simulink model "DualStreamSSR"  (R2023a)
(part 5 of 6)

  filter6 : aieBasic/AIE Class Kernel  KernelAllAttrs=|  PortNames={'sin1'; 'sin2'; 'cin'; 'cout'}  PortSerializedTypes={'{Q2{P{Tinput_stream{1{t{Scint16}}}}}}'; '{Q2{P{Tinput_stream{1{t{Scint16}}}}}}'; '{P{Tinput_stream{1{t{Scacc48_t}}}}}'; '{P{Toutput_stream{1{t{Scacc48_t}}}}}'}  PortWindowSizes={0.000000000000000000e+00; 0.000000000000000000e+00; 0.000000000000000000e+00; 0.000000000000000000e+00}  PortWindowMargins={0.000000000000000000e+00; 0.000000000000000000e+00; 0.000000000000000000e+00; 0.000000000000000000e+00}  PortSynchronicities={'auto', 'auto', 'auto', 'auto'}  PortSignalSizes={0.000000000000000000e+00; 0.000000000000000000e+00; 0.000000000000000000e+00; 8.000000000000000000e+00}  ClassTemplateSpecKind=implicit  ClassTemplateParamNames={'NSamples'; 'ShiftAcc'; 'DiscardSample'; 'SwapRead'}  ClassTemplateParamKinds={'nontype'; 'nontype'; 'nontype'; 'nontype'}  ClassTemplateParamTypes={'int'; 'int'; 'bool'; 'bool'}  ClassTemplateParamValues={'512', '15', '0', '0'}  ClassCtorParamNames={'taps'}  ClassCtorParamSerializedTypes={'{R{Q1{C{Scint16}4}}}'}  ClassCtorParamValues={'[146-91i 4086+5221i 237-54i -83-21i]'}  ClassIndex=1  ClassCtorIndex=1  ClassTabVisible=on  ClassTemplateParamsVisible=on  ClassCtorDeclVisible=on  ClassCtorParamsVisible=on  FunctionTabVisible=on  FunctionDecl=|  PortAttrs={ 'input', 'sin1', 'input_stream_cint16 * restrict', '', '', '', ''; 'input', 'sin2', 'input_stream_cint16 * restrict', '', '', '', ''; 'input', 'cin', 'input_stream< cacc48_t > *', '', '', '', ''; 'output', 'cout', 'output_stream< cacc48_t > *', '', '', '', 'OUTPUT_SIZE' }  PortAttrsEnables={'off', 'off', 'off', 'off', 'off', 'off', 'off';'off', 'off', 'off', 'off', 'off', 'off', 'off';'off', 'off', 'off', 'off', 'off', 'off', 'off';'off', 'off', 'off', 'off', 'off', 'off', 'on'}  SampleTime=-1  ClassDeclTypeOptions=|  ClassDecl=|  ClassTemplateParams={ 'NSamples', 'int', 'BURST_LENGTH'; 'ShiftAcc', 'int', 'SHIFT_ACC'; 'DiscardSample', 'bool', 'FALSE'; 'SwapRead', 'bool', 'FALSE' }  ClassTemplateParamsEnables={'off', 'off', 'on';'off', 'off', 'on';'off', 'off', 'on';'off', 'off', 'on'}  ClassCtorDeclTypeOptions=C[1 1]@t54@FIR_MultiKernel_cincout(cint16 const ( & taps ) [ 4 ])  ClassCtorDecl=FIR_MultiKernel_cincout(cint16 const ( & taps ) [ 4 ])  ClassCtorParams={ 'taps', 'cint16 const ( &) [ 4 ]', 'phi_6' }  KernelHeaderFile=FirDoubleStream.h  KernelClassName=DoubleStream::FIR_MultiKernel_cincout  KernelFunction=filter  KernelSourceFile=FirDoubleStream.cpp  KernelSearchPaths={'$SRC/aie_kernels'}  PreProcOptions={}  blockJsonConstraints="{\"type\":\"constraint\",\"constraintType\":\"location_kernel\",\"sid\":\"845\",\"lhs\":{\"type\":\"location\",\"templParam\":\"kernel\",\"args\":{\"type\":\"kernel\",\"name\":\"DualStreamSSR/SSR8/filter6\",\"sid\":\"845\"}},\"rhs\":{\"type\":\"tile\",\"args\":[{\"type\":\"evaluable\",\"expr\":\"29\",\"value\":29},{\"type\":\"evaluable\",\"expr\":\"0\",\"value\":0}]},\"equality\":true}"
      KernelAllAttrs=|
      | s[12;12;9;9;19;14;21;23;24;21;12;24;26;26;26;27;28;9;21;23;23;23;24;25;14;19;19;29]@FunctionNameDeclFileNamePortNamesPortTypesPortSerializedTypesPortDirectionsPortWindowSizeEnablesPortWindowMarginEnablesPortSynchronicityEnablesPortSignalSizeEnablesFunctionDeclFunctionTemplateSpecKindFunctionTemplateParamNamesFunctionTemplateParamKindsFunctionTemplateParamTypesFunctionTemplateParamValuesFunctionTemplateParamEnablesClassDeclClassTemplateSpecKindClassTemplateParamNamesClassTemplateParamKindsClassTemplateParamTypesClassTemplateParamValuesClassTemplateParamEnablesClassCtorDeclsClassCtorParamNamesClassCtorParamTypesClassCtorParamSerializedTypes[1 1]@C[28 1]@t6@filtert42@../../../aie/aie_kernels/FirDoubleStream.hC[4 1]@t4@sin1t4@sin2t3@cint4@coutC[4 1]@t30@input_stream_cint16 * restrictt30@input_stream_cint16 * restrictt26@input_stream< cacc48_t > *t27@output_stream< cacc48_t > *C[4 1]@t37@{Q2{P{Tinput_stream{1{t{Scint16}}}}}}t37@{Q2{P{Tinput_stream{1{t{Scint16}}}}}}t35@{P{Tinput_stream{1{t{Scacc48_t}}}}}t36@{P{Toutput_stream{1{t{Scacc48_t}}}}}C[4 1]@t5@inputt5@inputt5@inputt6@outputC[4 1]@l0@l0@l0@l0@C[4 1]@l0@l0@l0@l0@C[4 1]@l0@l0@l0@l0@C[4 1]@l0@l0@l0@l1@t281@namespace DoubleStream {
      | template < int NSamples, int ShiftAcc, bool DiscardSample, bool SwapRead > 
      | void FIR_MultiKernel_cincout::
      | filter(input_stream_cint16 * restrict sin1, input_stream_cint16 * restrict sin2, input_stream< cacc48_t > * cin, output_stream< cacc48_t > * cout);
      | }t4@nonee[0 1]@e[0 1]@e[0 1]@e[0 1]@e[0 1]@t132@namespace DoubleStream {
      | template < int NSamples, int ShiftAcc, bool DiscardSample, bool SwapRead > class FIR_MultiKernel_cincout;
      | }t8@implicitC[4 1]@t8@NSamplest8@ShiftAcct13@DiscardSamplet8@SwapReadC[4 1]@t7@nontypet7@nontypet7@nontypet7@nontypeC[4 1]@t3@intt3@intt4@boolt4@boolC[4 1]@nnnnC[4 1]@l1@l1@l1@l1@C[1 1]@t54@FIR_MultiKernel_cincout(cint16 const ( & taps ) [ 4 ])C[1 1]@C[1 1]@t4@tapsC[1 1]@C[1 1]@t23@cint16 const ( &) [ 4 ]C[1 1]@C[1 1]@t20@{R{Q1{C{Scint16}4}}}
      FunctionDecl=|
      | namespace DoubleStream {
      | template < int NSamples, int ShiftAcc, bool DiscardSample, bool SwapRead > 
      | void FIR_MultiKernel_cincout::
      | filter(input_stream_cint16 * restrict sin1, input_stream_cint16 * restrict sin2, input_stream< cacc48_t > * cin, output_stream< cacc48_t > * cout);
      | }
      ClassDeclTypeOptions=|
      | C[1 1]@t132@namespace DoubleStream {
      | template < int NSamples, int ShiftAcc, bool DiscardSample, bool SwapRead > class FIR_MultiKernel_cincout;
      | }
      ClassDecl=|
      | namespace DoubleStream {
      | template < int NSamples, int ShiftAcc, bool DiscardSample, bool SwapRead > class FIR_MultiKernel_cincout;
      | }
  filter60 : aieBasic/AIE Class Kernel  KernelAllAttrs=|  PortNames={'sin1'; 'sin2'; 'cin'; 'cout'}  PortSerializedTypes={'{Q2{P{Tinput_stream{1{t{Scint16}}}}}}'; '{Q2{P{Tinput_stream{1{t{Scint16}}}}}}'; '{P{Tinput_stream{1{t{Scacc48_t}}}}}'; '{P{Toutput_stream{1{t{Scacc48_t}}}}}'}  PortWindowSizes={0.000000000000000000e+00; 0.000000000000000000e+00; 0.000000000000000000e+00; 0.000000000000000000e+00}  PortWindowMargins={0.000000000000000000e+00; 0.000000000000000000e+00; 0.000000000000000000e+00; 0.000000000000000000e+00}  PortSynchronicities={'auto', 'auto', 'auto', 'auto'}  PortSignalSizes={0.000000000000000000e+00; 0.000000000000000000e+00; 0.000000000000000000e+00; 8.000000000000000000e+00}  ClassTemplateSpecKind=implicit  ClassTemplateParamNames={'NSamples'; 'ShiftAcc'; 'DiscardSample'; 'SwapRead'}  ClassTemplateParamKinds={'nontype'; 'nontype'; 'nontype'; 'nontype'}  ClassTemplateParamTypes={'int'; 'int'; 'bool'; 'bool'}  ClassTemplateParamValues={'512', '15', '0', '0'}  ClassCtorParamNames={'taps'}  ClassCtorParamSerializedTypes={'{R{Q1{C{Scint16}4}}}'}  ClassCtorParamValues={'[-21+26i 1183+239i 248-2878i -160+111i]'}  ClassIndex=1  ClassCtorIndex=1  ClassTabVisible=on  ClassTemplateParamsVisible=on  ClassCtorDeclVisible=on  ClassCtorParamsVisible=on  FunctionTabVisible=on  FunctionDecl=|  PortAttrs={ 'input', 'sin1', 'input_stream_cint16 * restrict', '', '', '', ''; 'input', 'sin2', 'input_stream_cint16 * restrict', '', '', '', ''; 'input', 'cin', 'input_stream< cacc48_t > *', '', '', '', ''; 'output', 'cout', 'output_stream< cacc48_t > *', '', '', '', 'OUTPUT_SIZE' }  PortAttrsEnables={'off', 'off', 'off', 'off', 'off', 'off', 'off';'off', 'off', 'off', 'off', 'off', 'off', 'off';'off', 'off', 'off', 'off', 'off', 'off', 'off';'off', 'off', 'off', 'off', 'off', 'off', 'on'}  SampleTime=-1  ClassDeclTypeOptions=|  ClassDecl=|  ClassTemplateParams={ 'NSamples', 'int', 'BURST_LENGTH'; 'ShiftAcc', 'int', 'SHIFT_ACC'; 'DiscardSample', 'bool', 'FALSE'; 'SwapRead', 'bool', 'FALSE' }  ClassTemplateParamsEnables={'off', 'off', 'on';'off', 'off', 'on';'off', 'off', 'on';'off', 'off', 'on'}  ClassCtorDeclTypeOptions=C[1 1]@t54@FIR_MultiKernel_cincout(cint16 const ( & taps ) [ 4 ])  ClassCtorDecl=FIR_MultiKernel_cincout(cint16 const ( & taps ) [ 4 ])  ClassCtorParams={ 'taps', 'cint16 const ( &) [ 4 ]', 'phi_2' }  KernelHeaderFile=FirDoubleStream.h  KernelClassName=DoubleStream::FIR_MultiKernel_cincout  KernelFunction=filter  KernelSourceFile=FirDoubleStream.cpp  KernelSearchPaths={'$SRC/aie_kernels'}  PreProcOptions={}  blockJsonConstraints="{\"type\":\"constraint\",\"constraintType\":\"location_kernel\",\"sid\":\"846\",\"lhs\":{\"type\":\"location\",\"templParam\":\"kernel\",\"args\":{\"type\":\"kernel\",\"name\":\"DualStreamSSR/SSR8/filter60\",\"sid\":\"846\"}},\"rhs\":{\"type\":\"tile\",\"args\":[{\"type\":\"evaluable\",\"expr\":\"29\",\"value\":29},{\"type\":\"evaluable\",\"expr\":\"4\",\"value\":4}]},\"equality\":true}"
      KernelAllAttrs=|
      | s[12;12;9;9;19;14;21;23;24;21;12;24;26;26;26;27;28;9;21;23;23;23;24;25;14;19;19;29]@FunctionNameDeclFileNamePortNamesPortTypesPortSerializedTypesPortDirectionsPortWindowSizeEnablesPortWindowMarginEnablesPortSynchronicityEnablesPortSignalSizeEnablesFunctionDeclFunctionTemplateSpecKindFunctionTemplateParamNamesFunctionTemplateParamKindsFunctionTemplateParamTypesFunctionTemplateParamValuesFunctionTemplateParamEnablesClassDeclClassTemplateSpecKindClassTemplateParamNamesClassTemplateParamKindsClassTemplateParamTypesClassTemplateParamValuesClassTemplateParamEnablesClassCtorDeclsClassCtorParamNamesClassCtorParamTypesClassCtorParamSerializedTypes[1 1]@C[28 1]@t6@filtert42@../../../aie/aie_kernels/FirDoubleStream.hC[4 1]@t4@sin1t4@sin2t3@cint4@coutC[4 1]@t30@input_stream_cint16 * restrictt30@input_stream_cint16 * restrictt26@input_stream< cacc48_t > *t27@output_stream< cacc48_t > *C[4 1]@t37@{Q2{P{Tinput_stream{1{t{Scint16}}}}}}t37@{Q2{P{Tinput_stream{1{t{Scint16}}}}}}t35@{P{Tinput_stream{1{t{Scacc48_t}}}}}t36@{P{Toutput_stream{1{t{Scacc48_t}}}}}C[4 1]@t5@inputt5@inputt5@inputt6@outputC[4 1]@l0@l0@l0@l0@C[4 1]@l0@l0@l0@l0@C[4 1]@l0@l0@l0@l0@C[4 1]@l0@l0@l0@l1@t281@namespace DoubleStream {
      | template < int NSamples, int ShiftAcc, bool DiscardSample, bool SwapRead > 
      | void FIR_MultiKernel_cincout::
      | filter(input_stream_cint16 * restrict sin1, input_stream_cint16 * restrict sin2, input_stream< cacc48_t > * cin, output_stream< cacc48_t > * cout);
      | }t4@nonee[0 1]@e[0 1]@e[0 1]@e[0 1]@e[0 1]@t132@namespace DoubleStream {
      | template < int NSamples, int ShiftAcc, bool DiscardSample, bool SwapRead > class FIR_MultiKernel_cincout;
      | }t8@implicitC[4 1]@t8@NSamplest8@ShiftAcct13@DiscardSamplet8@SwapReadC[4 1]@t7@nontypet7@nontypet7@nontypet7@nontypeC[4 1]@t3@intt3@intt4@boolt4@boolC[4 1]@nnnnC[4 1]@l1@l1@l1@l1@C[1 1]@t54@FIR_MultiKernel_cincout(cint16 const ( & taps ) [ 4 ])C[1 1]@C[1 1]@t4@tapsC[1 1]@C[1 1]@t23@cint16 const ( &) [ 4 ]C[1 1]@C[1 1]@t20@{R{Q1{C{Scint16}4}}}
      FunctionDecl=|
      | namespace DoubleStream {
      | template < int NSamples, int ShiftAcc, bool DiscardSample, bool SwapRead > 
      | void FIR_MultiKernel_cincout::
      | filter(input_stream_cint16 * restrict sin1, input_stream_cint16 * restrict sin2, input_stream< cacc48_t > * cin, output_stream< cacc48_t > * cout);
      | }
      ClassDeclTypeOptions=|
      | C[1 1]@t132@namespace DoubleStream {
      | template < int NSamples, int ShiftAcc, bool DiscardSample, bool SwapRead > class FIR_MultiKernel_cincout;
      | }
      ClassDecl=|
      | namespace DoubleStream {
      | template < int NSamples, int ShiftAcc, bool DiscardSample, bool SwapRead > class FIR_MultiKernel_cincout;
      | }
  filter61 : aieBasic/AIE Class Kernel  KernelAllAttrs=|  PortNames={'sin1'; 'sin2'; 'cin'; 'sout1'; 'sout2'}  PortSerializedTypes={'{Q2{P{Tinput_stream{1{t{Scint16}}}}}}'; '{Q2{P{Tinput_stream{1{t{Scint16}}}}}}'; '{P{Tinput_stream{1{t{Scacc48_t}}}}}'; '{Q2{P{Toutput_stream{1{t{Scint16}}}}}}'; '{Q2{P{Toutput_stream{1{t{Scint16}}}}}}'}  PortWindowSizes={0.000000000000000000e+00; 0.000000000000000000e+00; 0.000000000000000000e+00; 0.000000000000000000e+00; 0.000000000000000000e+00}  PortWindowMargins={0.000000000000000000e+00; 0.000000000000000000e+00; 0.000000000000000000e+00; 0.000000000000000000e+00; 0.000000000000000000e+00}  PortSynchronicities={'auto', 'auto', 'auto', 'auto', 'auto'}  PortSignalSizes={0.000000000000000000e+00; 0.000000000000000000e+00; 0.000000000000000000e+00; 4.000000000000000000e+00; 4.000000000000000000e+00}  ClassTemplateSpecKind=implicit  ClassTemplateParamNames={'NSamples'; 'ShiftAcc'; 'DiscardSample'; 'SwapRead'}  ClassTemplateParamKinds={'nontype'; 'nontype'; 'nontype'; 'nontype'}  ClassTemplateParamTypes={'int'; 'int'; 'bool'; 'bool'}  ClassTemplateParamValues={'512', '15', '0', '0'}  ClassCtorParamNames={'taps'}  ClassCtorParamSerializedTypes={'{R{Q1{C{Scint16}4}}}'}  ClassCtorParamValues={'[14-121i 1454-497i 237+96i -121+233i]'}  ClassIndex=1  ClassCtorIndex=1  ClassTabVisible=on  ClassTemplateParamsVisible=on  ClassCtorDeclVisible=on  ClassCtorParamsVisible=on  FunctionTabVisible=on  FunctionDecl=|  PortAttrs={ 'input', 'sin1', 'input_stream_cint16 * restrict', '', '', '', ''; 'input', 'sin2', 'input_stream_cint16 * restrict', '', '', '', ''; 'input', 'cin', 'input_stream< cacc48_t > *', '', '', '', ''; 'output', 'sout1', 'output_stream_cint16 * restrict', '', '', '', 'OUTPUT_SIZE/2'; 'output', 'sout2', 'output_stream_cint16 * restrict', '', '', '', 'OUTPUT_SIZE/2' }  PortAttrsEnables={'off', 'off', 'off', 'off', 'off', 'off', 'off';'off', 'off', 'off', 'off', 'off', 'off', 'off';'off', 'off', 'off', 'off', 'off', 'off', 'off';'off', 'off', 'off', 'off', 'off', 'off', 'on';'off', 'off', 'off', 'off', 'off', 'off', 'on'}  SampleTime=-1  ClassDeclTypeOptions=|  ClassDecl=|  ClassTemplateParams={ 'NSamples', 'int', 'BURST_LENGTH'; 'ShiftAcc', 'int', 'SHIFT_ACC'; 'DiscardSample', 'bool', 'FALSE'; 'SwapRead', 'bool', 'FALSE' }  ClassTemplateParamsEnables={'off', 'off', 'on';'off', 'off', 'on';'off', 'off', 'on';'off', 'off', 'on'}  ClassCtorDeclTypeOptions=C[1 1]@t50@FIR_MultiKernel_cin(cint16 const ( & taps ) [ 4 ])  ClassCtorDecl=FIR_MultiKernel_cin(cint16 const ( & taps ) [ 4 ])  ClassCtorParams={ 'taps', 'cint16 const ( &) [ 4 ]', 'phi_3' }  KernelHeaderFile=FirDoubleStream.h  KernelClassName=DoubleStream::FIR_MultiKernel_cin  KernelFunction=filter  KernelSourceFile=FirDoubleStream.cpp  KernelSearchPaths={'$SRC/aie_kernels'}  PreProcOptions={}  blockJsonConstraints="{\"type\":\"constraint\",\"constraintType\":\"location_kernel\",\"sid\":\"847\",\"lhs\":{\"type\":\"location\",\"templParam\":\"kernel\",\"args\":{\"type\":\"kernel\",\"name\":\"DualStreamSSR/SSR8/filter61\",\"sid\":\"847\"}},\"rhs\":{\"type\":\"tile\",\"args\":[{\"type\":\"evaluable\",\"expr\":\"30\",\"value\":30},{\"type\":\"evaluable\",\"expr\":\"4\",\"value\":4}]},\"equality\":true}"
      KernelAllAttrs=|
      | s[12;12;9;9;19;14;21;23;24;21;12;24;26;26;26;27;28;9;21;23;23;23;24;25;14;19;19;29]@FunctionNameDeclFileNamePortNamesPortTypesPortSerializedTypesPortDirectionsPortWindowSizeEnablesPortWindowMarginEnablesPortSynchronicityEnablesPortSignalSizeEnablesFunctionDeclFunctionTemplateSpecKindFunctionTemplateParamNamesFunctionTemplateParamKindsFunctionTemplateParamTypesFunctionTemplateParamValuesFunctionTemplateParamEnablesClassDeclClassTemplateSpecKindClassTemplateParamNamesClassTemplateParamKindsClassTemplateParamTypesClassTemplateParamValuesClassTemplateParamEnablesClassCtorDeclsClassCtorParamNamesClassCtorParamTypesClassCtorParamSerializedTypes[1 1]@C[28 1]@t6@filtert42@../../../aie/aie_kernels/FirDoubleStream.hC[5 1]@t4@sin1t4@sin2t3@cint5@sout1t5@sout2C[5 1]@t30@input_stream_cint16 * restrictt30@input_stream_cint16 * restrictt26@input_stream< cacc48_t > *t31@output_stream_cint16 * restrictt31@output_stream_cint16 * restrictC[5 1]@t37@{Q2{P{Tinput_stream{1{t{Scint16}}}}}}t37@{Q2{P{Tinput_stream{1{t{Scint16}}}}}}t35@{P{Tinput_stream{1{t{Scacc48_t}}}}}t38@{Q2{P{Toutput_stream{1{t{Scint16}}}}}}t38@{Q2{P{Toutput_stream{1{t{Scint16}}}}}}C[5 1]@t5@inputt5@inputt5@inputt6@outputt6@outputC[5 1]@l0@l0@l0@l0@l0@C[5 1]@l0@l0@l0@l0@l0@C[5 1]@l0@l0@l0@l0@l0@C[5 1]@l0@l0@l0@l1@l1@t321@namespace DoubleStream {
      | template < int NSamples, int ShiftAcc, bool DiscardSample, bool SwapRead > 
      | void FIR_MultiKernel_cin::
      | filter(input_stream_cint16 * restrict sin1, input_stream_cint16 * restrict sin2, input_stream< cacc48_t > * cin, output_stream_cint16 * restrict sout1, output_stream_cint16 * restrict sout2);
      | }t4@nonee[0 1]@e[0 1]@e[0 1]@e[0 1]@e[0 1]@t128@namespace DoubleStream {
      | template < int NSamples, int ShiftAcc, bool DiscardSample, bool SwapRead > class FIR_MultiKernel_cin;
      | }t8@implicitC[4 1]@t8@NSamplest8@ShiftAcct13@DiscardSamplet8@SwapReadC[4 1]@t7@nontypet7@nontypet7@nontypet7@nontypeC[4 1]@t3@intt3@intt4@boolt4@boolC[4 1]@nnnnC[4 1]@l1@l1@l1@l1@C[1 1]@t50@FIR_MultiKernel_cin(cint16 const ( & taps ) [ 4 ])C[1 1]@C[1 1]@t4@tapsC[1 1]@C[1 1]@t23@cint16 const ( &) [ 4 ]C[1 1]@C[1 1]@t20@{R{Q1{C{Scint16}4}}}
      FunctionDecl=|
      | namespace DoubleStream {
      | template < int NSamples, int ShiftAcc, bool DiscardSample, bool SwapRead > 
      | void FIR_MultiKernel_cin::
      | filter(input_stream_cint16 * restrict sin1, input_stream_cint16 * restrict sin2, input_stream< cacc48_t > * cin, output_stream_cint16 * restrict sout1, output_stream_cint16 * restrict sout2);
      | }
      ClassDeclTypeOptions=|
      | C[1 1]@t128@namespace DoubleStream {
      | template < int NSamples, int ShiftAcc, bool DiscardSample, bool SwapRead > class FIR_MultiKernel_cin;
      | }
      ClassDecl=|
      | namespace DoubleStream {
      | template < int NSamples, int ShiftAcc, bool DiscardSample, bool SwapRead > class FIR_MultiKernel_cin;
      | }
  filter62 : aieBasic/AIE Class Kernel  KernelAllAttrs=|  PortNames={'sin1'; 'sin2'; 'cout'}  PortSerializedTypes={'{Q2{P{Tinput_stream{1{t{Scint16}}}}}}'; '{Q2{P{Tinput_stream{1{t{Scint16}}}}}}'; '{P{Toutput_stream{1{t{Scacc48_t}}}}}'}  PortWindowSizes={0.000000000000000000e+00; 0.000000000000000000e+00; 0.000000000000000000e+00}  PortWindowMargins={0.000000000000000000e+00; 0.000000000000000000e+00; 0.000000000000000000e+00}  PortSynchronicities={'auto', 'auto', 'auto'}  PortSignalSizes={0.000000000000000000e+00; 0.000000000000000000e+00; 8.000000000000000000e+00}  ClassTemplateSpecKind=implicit  ClassTemplateParamNames={'NSamples'; 'ShiftAcc'; 'DiscardSample'; 'SwapRead'}  ClassTemplateParamKinds={'nontype'; 'nontype'; 'nontype'; 'nontype'}  ClassTemplateParamTypes={'int'; 'int'; 'bool'; 'bool'}  ClassTemplateParamValues={'512', '15', '0', '0'}  ClassCtorParamNames={'taps'}  ClassCtorParamSerializedTypes={'{R{Q1{C{Scint16}4}}}'}  ClassCtorParamValues={'[-21+26i 1183+239i 248-2878i -160+111i]'}  ClassIndex=1  ClassCtorIndex=1  ClassTabVisible=on  ClassTemplateParamsVisible=on  ClassCtorDeclVisible=on  ClassCtorParamsVisible=on  FunctionTabVisible=on  FunctionDecl=|  PortAttrs={ 'input', 'sin1', 'input_stream_cint16 * restrict', '', '', '', ''; 'input', 'sin2', 'input_stream_cint16 * restrict', '', '', '', ''; 'output', 'cout', 'output_stream< cacc48_t > *', '', '', '', 'OUTPUT_SIZE' }  PortAttrsEnables={'off', 'off', 'off', 'off', 'off', 'off', 'off';'off', 'off', 'off', 'off', 'off', 'off', 'off';'off', 'off', 'off', 'off', 'off', 'off', 'on'}  SampleTime=-1  ClassDeclTypeOptions=|  ClassDecl=|  ClassTemplateParams={ 'NSamples', 'int', 'BURST_LENGTH'; 'ShiftAcc', 'int', 'SHIFT_ACC'; 'DiscardSample', 'bool', 'FALSE'; 'SwapRead', 'bool', 'FALSE' }  ClassTemplateParamsEnables={'off', 'off', 'on';'off', 'off', 'on';'off', 'off', 'on';'off', 'off', 'on'}  ClassCtorDeclTypeOptions=C[1 1]@t51@FIR_MultiKernel_cout(cint16 const ( & taps ) [ 4 ])  ClassCtorDecl=FIR_MultiKernel_cout(cint16 const ( & taps ) [ 4 ])  ClassCtorParams={ 'taps', 'cint16 const ( &) [ 4 ]', 'phi_2' }  KernelHeaderFile=FirDoubleStream.h  KernelClassName=DoubleStream::FIR_MultiKernel_cout  KernelFunction=filter  KernelSourceFile=FirDoubleStream.cpp  KernelSearchPaths={'$SRC/aie_kernels'}  PreProcOptions={}  blockJsonConstraints="{\"type\":\"constraint\",\"constraintType\":\"location_kernel\",\"sid\":\"848\",\"lhs\":{\"type\":\"location\",\"templParam\":\"kernel\",\"args\":{\"type\":\"kernel\",\"name\":\"DualStreamSSR/SSR8/filter62\",\"sid\":\"848\"}},\"rhs\":{\"type\":\"tile\",\"args\":[{\"type\":\"evaluable\",\"expr\":\"30\",\"value\":30},{\"type\":\"evaluable\",\"expr\":\"5\",\"value\":5}]},\"equality\":true}"
      KernelAllAttrs=|
      | s[12;12;9;9;19;14;21;23;24;21;12;24;26;26;26;27;28;9;21;23;23;23;24;25;14;19;19;29]@FunctionNameDeclFileNamePortNamesPortTypesPortSerializedTypesPortDirectionsPortWindowSizeEnablesPortWindowMarginEnablesPortSynchronicityEnablesPortSignalSizeEnablesFunctionDeclFunctionTemplateSpecKindFunctionTemplateParamNamesFunctionTemplateParamKindsFunctionTemplateParamTypesFunctionTemplateParamValuesFunctionTemplateParamEnablesClassDeclClassTemplateSpecKindClassTemplateParamNamesClassTemplateParamKindsClassTemplateParamTypesClassTemplateParamValuesClassTemplateParamEnablesClassCtorDeclsClassCtorParamNamesClassCtorParamTypesClassCtorParamSerializedTypes[1 1]@C[28 1]@t6@filtert42@../../../aie/aie_kernels/FirDoubleStream.hC[3 1]@t4@sin1t4@sin2t4@coutC[3 1]@t30@input_stream_cint16 * restrictt30@input_stream_cint16 * restrictt27@output_stream< cacc48_t > *C[3 1]@t37@{Q2{P{Tinput_stream{1{t{Scint16}}}}}}t37@{Q2{P{Tinput_stream{1{t{Scint16}}}}}}t36@{P{Toutput_stream{1{t{Scacc48_t}}}}}C[3 1]@t5@inputt5@inputt6@outputC[3 1]@l0@l0@l0@C[3 1]@l0@l0@l0@C[3 1]@l0@l0@l0@C[3 1]@l0@l0@l1@t246@namespace DoubleStream {
      | template < int NSamples, int ShiftAcc, bool DiscardSample, bool SwapRead > 
      | void FIR_MultiKernel_cout::
      | filter(input_stream_cint16 * restrict sin1, input_stream_cint16 * restrict sin2, output_stream< cacc48_t > * cout);
      | }t4@nonee[0 1]@e[0 1]@e[0 1]@e[0 1]@e[0 1]@t129@namespace DoubleStream {
      | template < int NSamples, int ShiftAcc, bool DiscardSample, bool SwapRead > class FIR_MultiKernel_cout;
      | }t8@implicitC[4 1]@t8@NSamplest8@ShiftAcct13@DiscardSamplet8@SwapReadC[4 1]@t7@nontypet7@nontypet7@nontypet7@nontypeC[4 1]@t3@intt3@intt4@boolt4@boolC[4 1]@nnnnC[4 1]@l1@l1@l1@l1@C[1 1]@t51@FIR_MultiKernel_cout(cint16 const ( & taps ) [ 4 ])C[1 1]@C[1 1]@t4@tapsC[1 1]@C[1 1]@t23@cint16 const ( &) [ 4 ]C[1 1]@C[1 1]@t20@{R{Q1{C{Scint16}4}}}
      FunctionDecl=|
      | namespace DoubleStream {
      | template < int NSamples, int ShiftAcc, bool DiscardSample, bool SwapRead > 
      | void FIR_MultiKernel_cout::
      | filter(input_stream_cint16 * restrict sin1, input_stream_cint16 * restrict sin2, output_stream< cacc48_t > * cout);
      | }
      ClassDeclTypeOptions=|
      | C[1 1]@t129@namespace DoubleStream {
      | template < int NSamples, int ShiftAcc, bool DiscardSample, bool SwapRead > class FIR_MultiKernel_cout;
      | }
      ClassDecl=|
      | namespace DoubleStream {
      | template < int NSamples, int ShiftAcc, bool DiscardSample, bool SwapRead > class FIR_MultiKernel_cout;
      | }
  filter63 : aieBasic/AIE Class Kernel  KernelAllAttrs=|  PortNames={'sin1'; 'sin2'; 'cin'; 'cout'}  PortSerializedTypes={'{Q2{P{Tinput_stream{1{t{Scint16}}}}}}'; '{Q2{P{Tinput_stream{1{t{Scint16}}}}}}'; '{P{Tinput_stream{1{t{Scacc48_t}}}}}'; '{P{Toutput_stream{1{t{Scacc48_t}}}}}'}  PortWindowSizes={0.000000000000000000e+00; 0.000000000000000000e+00; 0.000000000000000000e+00; 0.000000000000000000e+00}  PortWindowMargins={0.000000000000000000e+00; 0.000000000000000000e+00; 0.000000000000000000e+00; 0.000000000000000000e+00}  PortSynchronicities={'auto', 'auto', 'auto', 'auto'}  PortSignalSizes={0.000000000000000000e+00; 0.000000000000000000e+00; 0.000000000000000000e+00; 8.000000000000000000e+00}  ClassTemplateSpecKind=implicit  ClassTemplateParamNames={'NSamples'; 'ShiftAcc'; 'DiscardSample'; 'SwapRead'}  ClassTemplateParamKinds={'nontype'; 'nontype'; 'nontype'; 'nontype'}  ClassTemplateParamTypes={'int'; 'int'; 'bool'; 'bool'}  ClassTemplateParamValues={'512', '15', '0', '0'}  ClassCtorParamNames={'taps'}  ClassCtorParamSerializedTypes={'{R{Q1{C{Scint16}4}}}'}  ClassCtorParamValues={'[-83+21i 237+54i 4086-5221i 146+91i]'}  ClassIndex=1  ClassCtorIndex=1  ClassTabVisible=on  ClassTemplateParamsVisible=on  ClassCtorDeclVisible=on  ClassCtorParamsVisible=on  FunctionTabVisible=on  FunctionDecl=|  PortAttrs={ 'input', 'sin1', 'input_stream_cint16 * restrict', '', '', '', ''; 'input', 'sin2', 'input_stream_cint16 * restrict', '', '', '', ''; 'input', 'cin', 'input_stream< cacc48_t > *', '', '', '', ''; 'output', 'cout', 'output_stream< cacc48_t > *', '', '', '', 'OUTPUT_SIZE' }  PortAttrsEnables={'off', 'off', 'off', 'off', 'off', 'off', 'off';'off', 'off', 'off', 'off', 'off', 'off', 'off';'off', 'off', 'off', 'off', 'off', 'off', 'off';'off', 'off', 'off', 'off', 'off', 'off', 'on'}  SampleTime=-1  ClassDeclTypeOptions=|  ClassDecl=|  ClassTemplateParams={ 'NSamples', 'int', 'BURST_LENGTH'; 'ShiftAcc', 'int', 'SHIFT_ACC'; 'DiscardSample', 'bool', 'FALSE'; 'SwapRead', 'bool', 'FALSE' }  ClassTemplateParamsEnables={'off', 'off', 'on';'off', 'off', 'on';'off', 'off', 'on';'off', 'off', 'on'}  ClassCtorDeclTypeOptions=C[1 1]@t54@FIR_MultiKernel_cincout(cint16 const ( & taps ) [ 4 ])  ClassCtorDecl=FIR_MultiKernel_cincout(cint16 const ( & taps ) [ 4 ])  ClassCtorParams={ 'taps', 'cint16 const ( &) [ 4 ]', 'phi_1' }  KernelHeaderFile=FirDoubleStream.h  KernelClassName=DoubleStream::FIR_MultiKernel_cincout  KernelFunction=filter  KernelSourceFile=FirDoubleStream.cpp  KernelSearchPaths={'$SRC/aie_kernels'}  PreProcOptions={}  blockJsonConstraints="{\"type\":\"constraint\",\"constraintType\":\"location_kernel\",\"sid\":\"849\",\"lhs\":{\"type\":\"location\",\"templParam\":\"kernel\",\"args\":{\"type\":\"kernel\",\"name\":\"DualStreamSSR/SSR8/filter63\",\"sid\":\"849\"}},\"rhs\":{\"type\":\"tile\",\"args\":[{\"type\":\"evaluable\",\"expr\":\"29\",\"value\":29},{\"type\":\"evaluable\",\"expr\":\"5\",\"value\":5}]},\"equality\":true}"
      KernelAllAttrs=|
      | s[12;12;9;9;19;14;21;23;24;21;12;24;26;26;26;27;28;9;21;23;23;23;24;25;14;19;19;29]@FunctionNameDeclFileNamePortNamesPortTypesPortSerializedTypesPortDirectionsPortWindowSizeEnablesPortWindowMarginEnablesPortSynchronicityEnablesPortSignalSizeEnablesFunctionDeclFunctionTemplateSpecKindFunctionTemplateParamNamesFunctionTemplateParamKindsFunctionTemplateParamTypesFunctionTemplateParamValuesFunctionTemplateParamEnablesClassDeclClassTemplateSpecKindClassTemplateParamNamesClassTemplateParamKindsClassTemplateParamTypesClassTemplateParamValuesClassTemplateParamEnablesClassCtorDeclsClassCtorParamNamesClassCtorParamTypesClassCtorParamSerializedTypes[1 1]@C[28 1]@t6@filtert42@../../../aie/aie_kernels/FirDoubleStream.hC[4 1]@t4@sin1t4@sin2t3@cint4@coutC[4 1]@t30@input_stream_cint16 * restrictt30@input_stream_cint16 * restrictt26@input_stream< cacc48_t > *t27@output_stream< cacc48_t > *C[4 1]@t37@{Q2{P{Tinput_stream{1{t{Scint16}}}}}}t37@{Q2{P{Tinput_stream{1{t{Scint16}}}}}}t35@{P{Tinput_stream{1{t{Scacc48_t}}}}}t36@{P{Toutput_stream{1{t{Scacc48_t}}}}}C[4 1]@t5@inputt5@inputt5@inputt6@outputC[4 1]@l0@l0@l0@l0@C[4 1]@l0@l0@l0@l0@C[4 1]@l0@l0@l0@l0@C[4 1]@l0@l0@l0@l1@t281@namespace DoubleStream {
      | template < int NSamples, int ShiftAcc, bool DiscardSample, bool SwapRead > 
      | void FIR_MultiKernel_cincout::
      | filter(input_stream_cint16 * restrict sin1, input_stream_cint16 * restrict sin2, input_stream< cacc48_t > * cin, output_stream< cacc48_t > * cout);
      | }t4@nonee[0 1]@e[0 1]@e[0 1]@e[0 1]@e[0 1]@t132@namespace DoubleStream {
      | template < int NSamples, int ShiftAcc, bool DiscardSample, bool SwapRead > class FIR_MultiKernel_cincout;
      | }t8@implicitC[4 1]@t8@NSamplest8@ShiftAcct13@DiscardSamplet8@SwapReadC[4 1]@t7@nontypet7@nontypet7@nontypet7@nontypeC[4 1]@t3@intt3@intt4@boolt4@boolC[4 1]@nnnnC[4 1]@l1@l1@l1@l1@C[1 1]@t54@FIR_MultiKernel_cincout(cint16 const ( & taps ) [ 4 ])C[1 1]@C[1 1]@t4@tapsC[1 1]@C[1 1]@t23@cint16 const ( &) [ 4 ]C[1 1]@C[1 1]@t20@{R{Q1{C{Scint16}4}}}
      FunctionDecl=|
      | namespace DoubleStream {
      | template < int NSamples, int ShiftAcc, bool DiscardSample, bool SwapRead > 
      | void FIR_MultiKernel_cincout::
      | filter(input_stream_cint16 * restrict sin1, input_stream_cint16 * restrict sin2, input_stream< cacc48_t > * cin, output_stream< cacc48_t > * cout);
      | }
      ClassDeclTypeOptions=|
      | C[1 1]@t132@namespace DoubleStream {
      | template < int NSamples, int ShiftAcc, bool DiscardSample, bool SwapRead > class FIR_MultiKernel_cincout;
      | }
      ClassDecl=|
      | namespace DoubleStream {
      | template < int NSamples, int ShiftAcc, bool DiscardSample, bool SwapRead > class FIR_MultiKernel_cincout;
      | }
  filter7 : aieBasic/AIE Class Kernel  KernelAllAttrs=|  PortNames={'sin1'; 'sin2'; 'cin'; 'sout1'; 'sout2'}  PortSerializedTypes={'{Q2{P{Tinput_stream{1{t{Scint16}}}}}}'; '{Q2{P{Tinput_stream{1{t{Scint16}}}}}}'; '{P{Tinput_stream{1{t{Scacc48_t}}}}}'; '{Q2{P{Toutput_stream{1{t{Scint16}}}}}}'; '{Q2{P{Toutput_stream{1{t{Scint16}}}}}}'}  PortWindowSizes={0.000000000000000000e+00; 0.000000000000000000e+00; 0.000000000000000000e+00; 0.000000000000000000e+00; 0.000000000000000000e+00}  PortWindowMargins={0.000000000000000000e+00; 0.000000000000000000e+00; 0.000000000000000000e+00; 0.000000000000000000e+00; 0.000000000000000000e+00}  PortSynchronicities={'auto', 'auto', 'auto', 'auto', 'auto'}  PortSignalSizes={0.000000000000000000e+00; 0.000000000000000000e+00; 0.000000000000000000e+00; 4.000000000000000000e+00; 4.000000000000000000e+00}  ClassTemplateSpecKind=implicit  ClassTemplateParamNames={'NSamples'; 'ShiftAcc'; 'DiscardSample'; 'SwapRead'}  ClassTemplateParamKinds={'nontype'; 'nontype'; 'nontype'; 'nontype'}  ClassTemplateParamTypes={'int'; 'int'; 'bool'; 'bool'}  ClassTemplateParamValues={'512', '15', '0', '0'}  ClassCtorParamNames={'taps'}  ClassCtorParamSerializedTypes={'{R{Q1{C{Scint16}4}}}'}  ClassCtorParamValues={'[342-439i 8773+2748i 102+525i -54+21i]'}  ClassIndex=1  ClassCtorIndex=1  ClassTabVisible=on  ClassTemplateParamsVisible=on  ClassCtorDeclVisible=on  ClassCtorParamsVisible=on  FunctionTabVisible=on  FunctionDecl=|  PortAttrs={ 'input', 'sin1', 'input_stream_cint16 * restrict', '', '', '', ''; 'input', 'sin2', 'input_stream_cint16 * restrict', '', '', '', ''; 'input', 'cin', 'input_stream< cacc48_t > *', '', '', '', ''; 'output', 'sout1', 'output_stream_cint16 * restrict', '', '', '', 'OUTPUT_SIZE/2'; 'output', 'sout2', 'output_stream_cint16 * restrict', '', '', '', 'OUTPUT_SIZE/2' }  PortAttrsEnables={'off', 'off', 'off', 'off', 'off', 'off', 'off';'off', 'off', 'off', 'off', 'off', 'off', 'off';'off', 'off', 'off', 'off', 'off', 'off', 'off';'off', 'off', 'off', 'off', 'off', 'off', 'on';'off', 'off', 'off', 'off', 'off', 'off', 'on'}  SampleTime=-1  ClassDeclTypeOptions=|  ClassDecl=|  ClassTemplateParams={ 'NSamples', 'int', 'BURST_LENGTH'; 'ShiftAcc', 'int', 'SHIFT_ACC'; 'DiscardSample', 'bool', 'FALSE'; 'SwapRead', 'bool', 'FALSE' }  ClassTemplateParamsEnables={'off', 'off', 'on';'off', 'off', 'on';'off', 'off', 'on';'off', 'off', 'on'}  ClassCtorDeclTypeOptions=C[1 1]@t50@FIR_MultiKernel_cin(cint16 const ( & taps ) [ 4 ])  ClassCtorDecl=FIR_MultiKernel_cin(cint16 const ( & taps ) [ 4 ])  ClassCtorParams={ 'taps', 'cint16 const ( &) [ 4 ]', 'phi_7' }  KernelHeaderFile=FirDoubleStream.h  KernelClassName=DoubleStream::FIR_MultiKernel_cin  KernelFunction=filter  KernelSourceFile=FirDoubleStream.cpp  KernelSearchPaths={'$SRC/aie_kernels'}  PreProcOptions={}  blockJsonConstraints="{\"type\":\"constraint\",\"constraintType\":\"location_kernel\",\"sid\":\"850\",\"lhs\":{\"type\":\"location\",\"templParam\":\"kernel\",\"args\":{\"type\":\"kernel\",\"name\":\"DualStreamSSR/SSR8/filter7\",\"sid\":\"850\"}},\"rhs\":{\"type\":\"tile\",\"args\":[{\"type\":\"evaluable\",\"expr\":\"30\",\"value\":30},{\"type\":\"evaluable\",\"expr\":\"0\",\"value\":0}]},\"equality\":true}"
      KernelAllAttrs=|
      | s[12;12;9;9;19;14;21;23;24;21;12;24;26;26;26;27;28;9;21;23;23;23;24;25;14;19;19;29]@FunctionNameDeclFileNamePortNamesPortTypesPortSerializedTypesPortDirectionsPortWindowSizeEnablesPortWindowMarginEnablesPortSynchronicityEnablesPortSignalSizeEnablesFunctionDeclFunctionTemplateSpecKindFunctionTemplateParamNamesFunctionTemplateParamKindsFunctionTemplateParamTypesFunctionTemplateParamValuesFunctionTemplateParamEnablesClassDeclClassTemplateSpecKindClassTemplateParamNamesClassTemplateParamKindsClassTemplateParamTypesClassTemplateParamValuesClassTemplateParamEnablesClassCtorDeclsClassCtorParamNamesClassCtorParamTypesClassCtorParamSerializedTypes[1 1]@C[28 1]@t6@filtert42@../../../aie/aie_kernels/FirDoubleStream.hC[5 1]@t4@sin1t4@sin2t3@cint5@sout1t5@sout2C[5 1]@t30@input_stream_cint16 * restrictt30@input_stream_cint16 * restrictt26@input_stream< cacc48_t > *t31@output_stream_cint16 * restrictt31@output_stream_cint16 * restrictC[5 1]@t37@{Q2{P{Tinput_stream{1{t{Scint16}}}}}}t37@{Q2{P{Tinput_stream{1{t{Scint16}}}}}}t35@{P{Tinput_stream{1{t{Scacc48_t}}}}}t38@{Q2{P{Toutput_stream{1{t{Scint16}}}}}}t38@{Q2{P{Toutput_stream{1{t{Scint16}}}}}}C[5 1]@t5@inputt5@inputt5@inputt6@outputt6@outputC[5 1]@l0@l0@l0@l0@l0@C[5 1]@l0@l0@l0@l0@l0@C[5 1]@l0@l0@l0@l0@l0@C[5 1]@l0@l0@l0@l1@l1@t321@namespace DoubleStream {
      | template < int NSamples, int ShiftAcc, bool DiscardSample, bool SwapRead > 
      | void FIR_MultiKernel_cin::
      | filter(input_stream_cint16 * restrict sin1, input_stream_cint16 * restrict sin2, input_stream< cacc48_t > * cin, output_stream_cint16 * restrict sout1, output_stream_cint16 * restrict sout2);
      | }t4@nonee[0 1]@e[0 1]@e[0 1]@e[0 1]@e[0 1]@t128@namespace DoubleStream {
      | template < int NSamples, int ShiftAcc, bool DiscardSample, bool SwapRead > class FIR_MultiKernel_cin;
      | }t8@implicitC[4 1]@t8@NSamplest8@ShiftAcct13@DiscardSamplet8@SwapReadC[4 1]@t7@nontypet7@nontypet7@nontypet7@nontypeC[4 1]@t3@intt3@intt4@boolt4@boolC[4 1]@nnnnC[4 1]@l1@l1@l1@l1@C[1 1]@t50@FIR_MultiKernel_cin(cint16 const ( & taps ) [ 4 ])C[1 1]@C[1 1]@t4@tapsC[1 1]@C[1 1]@t23@cint16 const ( &) [ 4 ]C[1 1]@C[1 1]@t20@{R{Q1{C{Scint16}4}}}
      FunctionDecl=|
      | namespace DoubleStream {
      | template < int NSamples, int ShiftAcc, bool DiscardSample, bool SwapRead > 
      | void FIR_MultiKernel_cin::
      | filter(input_stream_cint16 * restrict sin1, input_stream_cint16 * restrict sin2, input_stream< cacc48_t > * cin, output_stream_cint16 * restrict sout1, output_stream_cint16 * restrict sout2);
      | }
      ClassDeclTypeOptions=|
      | C[1 1]@t128@namespace DoubleStream {
      | template < int NSamples, int ShiftAcc, bool DiscardSample, bool SwapRead > class FIR_MultiKernel_cin;
      | }
      ClassDecl=|
      | namespace DoubleStream {
      | template < int NSamples, int ShiftAcc, bool DiscardSample, bool SwapRead > class FIR_MultiKernel_cin;
      | }
  filter8 : aieBasic/AIE Class Kernel  KernelAllAttrs=|  PortNames={'sin1'; 'sin2'; 'cout'}  PortSerializedTypes={'{Q2{P{Tinput_stream{1{t{Scint16}}}}}}'; '{Q2{P{Tinput_stream{1{t{Scint16}}}}}}'; '{P{Toutput_stream{1{t{Scacc48_t}}}}}'}  PortWindowSizes={0.000000000000000000e+00; 0.000000000000000000e+00; 0.000000000000000000e+00}  PortWindowMargins={0.000000000000000000e+00; 0.000000000000000000e+00; 0.000000000000000000e+00}  PortSynchronicities={'auto', 'auto', 'auto'}  PortSignalSizes={0.000000000000000000e+00; 0.000000000000000000e+00; 8.000000000000000000e+00}  ClassTemplateSpecKind=implicit  ClassTemplateParamNames={'NSamples'; 'ShiftAcc'; 'DiscardSample'; 'SwapRead'}  ClassTemplateParamKinds={'nontype'; 'nontype'; 'nontype'; 'nontype'}  ClassTemplateParamTypes={'int'; 'int'; 'bool'; 'bool'}  ClassTemplateParamValues={'512', '15', '0', '0'}  ClassCtorParamNames={'taps'}  ClassCtorParamSerializedTypes={'{R{Q1{C{Scint16}4}}}'}  ClassCtorParamValues={'[146-91i 4086+5221i 237-54i -83-21i]'}  ClassIndex=1  ClassCtorIndex=1  ClassTabVisible=on  ClassTemplateParamsVisible=on  ClassCtorDeclVisible=on  ClassCtorParamsVisible=on  FunctionTabVisible=on  FunctionDecl=|  PortAttrs={ 'input', 'sin1', 'input_stream_cint16 * restrict', '', '', '', ''; 'input', 'sin2', 'input_stream_cint16 * restrict', '', '', '', ''; 'output', 'cout', 'output_stream< cacc48_t > *', '', '', '', 'OUTPUT_SIZE' }  PortAttrsEnables={'off', 'off', 'off', 'off', 'off', 'off', 'off';'off', 'off', 'off', 'off', 'off', 'off', 'off';'off', 'off', 'off', 'off', 'off', 'off', 'on'}  SampleTime=-1  ClassDeclTypeOptions=|  ClassDecl=|  ClassTemplateParams={ 'NSamples', 'int', 'BURST_LENGTH'; 'ShiftAcc', 'int', 'SHIFT_ACC'; 'DiscardSample', 'bool', 'FALSE'; 'SwapRead', 'bool', 'FALSE' }  ClassTemplateParamsEnables={'off', 'off', 'on';'off', 'off', 'on';'off', 'off', 'on';'off', 'off', 'on'}  ClassCtorDeclTypeOptions=C[1 1]@t51@FIR_MultiKernel_cout(cint16 const ( & taps ) [ 4 ])  ClassCtorDecl=FIR_MultiKernel_cout(cint16 const ( & taps ) [ 4 ])  ClassCtorParams={ 'taps', 'cint16 const ( &) [ 4 ]', 'phi_6' }  KernelHeaderFile=FirDoubleStream.h  KernelClassName=DoubleStream::FIR_MultiKernel_cout  KernelFunction=filter  KernelSourceFile=FirDoubleStream.cpp  KernelSearchPaths={'$SRC/aie_kernels'}  PreProcOptions={}  blockJsonConstraints="{\"type\":\"constraint\",\"constraintType\":\"location_kernel\",\"sid\":\"851\",\"lhs\":{\"type\":\"location\",\"templParam\":\"kernel\",\"args\":{\"type\":\"kernel\",\"name\":\"DualStreamSSR/SSR8/filter8\",\"sid\":\"851\"}},\"rhs\":{\"type\":\"tile\",\"args\":[{\"type\":\"evaluable\",\"expr\":\"30\",\"value\":30},{\"type\":\"evaluable\",\"expr\":\"1\",\"value\":1}]},\"equality\":true}"
      KernelAllAttrs=|
      | s[12;12;9;9;19;14;21;23;24;21;12;24;26;26;26;27;28;9;21;23;23;23;24;25;14;19;19;29]@FunctionNameDeclFileNamePortNamesPortTypesPortSerializedTypesPortDirectionsPortWindowSizeEnablesPortWindowMarginEnablesPortSynchronicityEnablesPortSignalSizeEnablesFunctionDeclFunctionTemplateSpecKindFunctionTemplateParamNamesFunctionTemplateParamKindsFunctionTemplateParamTypesFunctionTemplateParamValuesFunctionTemplateParamEnablesClassDeclClassTemplateSpecKindClassTemplateParamNamesClassTemplateParamKindsClassTemplateParamTypesClassTemplateParamValuesClassTemplateParamEnablesClassCtorDeclsClassCtorParamNamesClassCtorParamTypesClassCtorParamSerializedTypes[1 1]@C[28 1]@t6@filtert42@../../../aie/aie_kernels/FirDoubleStream.hC[3 1]@t4@sin1t4@sin2t4@coutC[3 1]@t30@input_stream_cint16 * restrictt30@input_stream_cint16 * restrictt27@output_stream< cacc48_t > *C[3 1]@t37@{Q2{P{Tinput_stream{1{t{Scint16}}}}}}t37@{Q2{P{Tinput_stream{1{t{Scint16}}}}}}t36@{P{Toutput_stream{1{t{Scacc48_t}}}}}C[3 1]@t5@inputt5@inputt6@outputC[3 1]@l0@l0@l0@C[3 1]@l0@l0@l0@C[3 1]@l0@l0@l0@C[3 1]@l0@l0@l1@t246@namespace DoubleStream {
      | template < int NSamples, int ShiftAcc, bool DiscardSample, bool SwapRead > 
      | void FIR_MultiKernel_cout::
      | filter(input_stream_cint16 * restrict sin1, input_stream_cint16 * restrict sin2, output_stream< cacc48_t > * cout);
      | }t4@nonee[0 1]@e[0 1]@e[0 1]@e[0 1]@e[0 1]@t129@namespace DoubleStream {
      | template < int NSamples, int ShiftAcc, bool DiscardSample, bool SwapRead > class FIR_MultiKernel_cout;
      | }t8@implicitC[4 1]@t8@NSamplest8@ShiftAcct13@DiscardSamplet8@SwapReadC[4 1]@t7@nontypet7@nontypet7@nontypet7@nontypeC[4 1]@t3@intt3@intt4@boolt4@boolC[4 1]@nnnnC[4 1]@l1@l1@l1@l1@C[1 1]@t51@FIR_MultiKernel_cout(cint16 const ( & taps ) [ 4 ])C[1 1]@C[1 1]@t4@tapsC[1 1]@C[1 1]@t23@cint16 const ( &) [ 4 ]C[1 1]@C[1 1]@t20@{R{Q1{C{Scint16}4}}}
      FunctionDecl=|
      | namespace DoubleStream {
      | template < int NSamples, int ShiftAcc, bool DiscardSample, bool SwapRead > 
      | void FIR_MultiKernel_cout::
      | filter(input_stream_cint16 * restrict sin1, input_stream_cint16 * restrict sin2, output_stream< cacc48_t > * cout);
      | }
      ClassDeclTypeOptions=|
      | C[1 1]@t129@namespace DoubleStream {
      | template < int NSamples, int ShiftAcc, bool DiscardSample, bool SwapRead > class FIR_MultiKernel_cout;
      | }
      ClassDecl=|
      | namespace DoubleStream {
      | template < int NSamples, int ShiftAcc, bool DiscardSample, bool SwapRead > class FIR_MultiKernel_cout;
      | }
  filter9 : aieBasic/AIE Class Kernel  KernelAllAttrs=|  PortNames={'sin1'; 'sin2'; 'cin'; 'cout'}  PortSerializedTypes={'{Q2{P{Tinput_stream{1{t{Scint16}}}}}}'; '{Q2{P{Tinput_stream{1{t{Scint16}}}}}}'; '{P{Tinput_stream{1{t{Scacc48_t}}}}}'; '{P{Toutput_stream{1{t{Scacc48_t}}}}}'}  PortWindowSizes={0.000000000000000000e+00; 0.000000000000000000e+00; 0.000000000000000000e+00; 0.000000000000000000e+00}  PortWindowMargins={0.000000000000000000e+00; 0.000000000000000000e+00; 0.000000000000000000e+00; 0.000000000000000000e+00}  PortSynchronicities={'auto', 'auto', 'auto', 'auto'}  PortSignalSizes={0.000000000000000000e+00; 0.000000000000000000e+00; 0.000000000000000000e+00; 8.000000000000000000e+00}  ClassTemplateSpecKind=implicit  ClassTemplateParamNames={'NSamples'; 'ShiftAcc'; 'DiscardSample'; 'SwapRead'}  ClassTemplateParamKinds={'nontype'; 'nontype'; 'nontype'; 'nontype'}  ClassTemplateParamTypes={'int'; 'int'; 'bool'; 'bool'}  ClassTemplateParamValues={'512', '15', '0', '0'}  ClassCtorParamNames={'taps'}  ClassCtorParamSerializedTypes={'{R{Q1{C{Scint16}4}}}'}  ClassCtorParamValues={'[-83+21i 237+54i 4086-5221i 146+91i]'}  ClassIndex=1  ClassCtorIndex=1  ClassTabVisible=on  ClassTemplateParamsVisible=on  ClassCtorDeclVisible=on  ClassCtorParamsVisible=on  FunctionTabVisible=on  FunctionDecl=|  PortAttrs={ 'input', 'sin1', 'input_stream_cint16 * restrict', '', '', '', ''; 'input', 'sin2', 'input_stream_cint16 * restrict', '', '', '', ''; 'input', 'cin', 'input_stream< cacc48_t > *', '', '', '', ''; 'output', 'cout', 'output_stream< cacc48_t > *', '', '', '', 'OUTPUT_SIZE' }  PortAttrsEnables={'off', 'off', 'off', 'off', 'off', 'off', 'off';'off', 'off', 'off', 'off', 'off', 'off', 'off';'off', 'off', 'off', 'off', 'off', 'off', 'off';'off', 'off', 'off', 'off', 'off', 'off', 'on'}  SampleTime=-1  ClassDeclTypeOptions=|  ClassDecl=|  ClassTemplateParams={ 'NSamples', 'int', 'BURST_LENGTH'; 'ShiftAcc', 'int', 'SHIFT_ACC'; 'DiscardSample', 'bool', 'FALSE'; 'SwapRead', 'bool', 'FALSE' }  ClassTemplateParamsEnables={'off', 'off', 'on';'off', 'off', 'on';'off', 'off', 'on';'off', 'off', 'on'}  ClassCtorDeclTypeOptions=C[1 1]@t54@FIR_MultiKernel_cincout(cint16 const ( & taps ) [ 4 ])  ClassCtorDecl=FIR_MultiKernel_cincout(cint16 const ( & taps ) [ 4 ])  ClassCtorParams={ 'taps', 'cint16 const ( &) [ 4 ]', 'phi_1' }  KernelHeaderFile=FirDoubleStream.h  KernelClassName=DoubleStream::FIR_MultiKernel_cincout  KernelFunction=filter  KernelSourceFile=FirDoubleStream.cpp  KernelSearchPaths={'$SRC/aie_kernels'}  PreProcOptions={}  blockJsonConstraints="{\"type\":\"constraint\",\"constraintType\":\"location_kernel\",\"sid\":\"852\",\"lhs\":{\"type\":\"location\",\"templParam\":\"kernel\",\"args\":{\"type\":\"kernel\",\"name\":\"DualStreamSSR/SSR8/filter9\",\"sid\":\"852\"}},\"rhs\":{\"type\":\"tile\",\"args\":[{\"type\":\"evaluable\",\"expr\":\"25\",\"value\":25},{\"type\":\"evaluable\",\"expr\":\"1\",\"value\":1}]},\"equality\":true}"
      KernelAllAttrs=|
      | s[12;12;9;9;19;14;21;23;24;21;12;24;26;26;26;27;28;9;21;23;23;23;24;25;14;19;19;29]@FunctionNameDeclFileNamePortNamesPortTypesPortSerializedTypesPortDirectionsPortWindowSizeEnablesPortWindowMarginEnablesPortSynchronicityEnablesPortSignalSizeEnablesFunctionDeclFunctionTemplateSpecKindFunctionTemplateParamNamesFunctionTemplateParamKindsFunctionTemplateParamTypesFunctionTemplateParamValuesFunctionTemplateParamEnablesClassDeclClassTemplateSpecKindClassTemplateParamNamesClassTemplateParamKindsClassTemplateParamTypesClassTemplateParamValuesClassTemplateParamEnablesClassCtorDeclsClassCtorParamNamesClassCtorParamTypesClassCtorParamSerializedTypes[1 1]@C[28 1]@t6@filtert42@../../../aie/aie_kernels/FirDoubleStream.hC[4 1]@t4@sin1t4@sin2t3@cint4@coutC[4 1]@t30@input_stream_cint16 * restrictt30@input_stream_cint16 * restrictt26@input_stream< cacc48_t > *t27@output_stream< cacc48_t > *C[4 1]@t37@{Q2{P{Tinput_stream{1{t{Scint16}}}}}}t37@{Q2{P{Tinput_stream{1{t{Scint16}}}}}}t35@{P{Tinput_stream{1{t{Scacc48_t}}}}}t36@{P{Toutput_stream{1{t{Scacc48_t}}}}}C[4 1]@t5@inputt5@inputt5@inputt6@outputC[4 1]@l0@l0@l0@l0@C[4 1]@l0@l0@l0@l0@C[4 1]@l0@l0@l0@l0@C[4 1]@l0@l0@l0@l1@t281@namespace DoubleStream {
      | template < int NSamples, int ShiftAcc, bool DiscardSample, bool SwapRead > 
      | void FIR_MultiKernel_cincout::
      | filter(input_stream_cint16 * restrict sin1, input_stream_cint16 * restrict sin2, input_stream< cacc48_t > * cin, output_stream< cacc48_t > * cout);
      | }t4@nonee[0 1]@e[0 1]@e[0 1]@e[0 1]@e[0 1]@t132@namespace DoubleStream {
      | template < int NSamples, int ShiftAcc, bool DiscardSample, bool SwapRead > class FIR_MultiKernel_cincout;
      | }t8@implicitC[4 1]@t8@NSamplest8@ShiftAcct13@DiscardSamplet8@SwapReadC[4 1]@t7@nontypet7@nontypet7@nontypet7@nontypeC[4 1]@t3@intt3@intt4@boolt4@boolC[4 1]@nnnnC[4 1]@l1@l1@l1@l1@C[1 1]@t54@FIR_MultiKernel_cincout(cint16 const ( & taps ) [ 4 ])C[1 1]@C[1 1]@t4@tapsC[1 1]@C[1 1]@t23@cint16 const ( &) [ 4 ]C[1 1]@C[1 1]@t20@{R{Q1{C{Scint16}4}}}
      FunctionDecl=|
      | namespace DoubleStream {
      | template < int NSamples, int ShiftAcc, bool DiscardSample, bool SwapRead > 
      | void FIR_MultiKernel_cincout::
      | filter(input_stream_cint16 * restrict sin1, input_stream_cint16 * restrict sin2, input_stream< cacc48_t > * cin, output_stream< cacc48_t > * cout);
      | }
      ClassDeclTypeOptions=|
      | C[1 1]@t132@namespace DoubleStream {
      | template < int NSamples, int ShiftAcc, bool DiscardSample, bool SwapRead > class FIR_MultiKernel_cincout;
      | }
      ClassDecl=|
      | namespace DoubleStream {
      | template < int NSamples, int ShiftAcc, bool DiscardSample, bool SwapRead > class FIR_MultiKernel_cincout;
      | }
  Phase0_out0 : Outport
  Phase0_out1 : Outport  Port=2
  Phase1_out0 : Outport  Port=3
  Phase1_out1 : Outport  Port=4
  Phase2_out0 : Outport  Port=5
  Phase2_out1 : Outport  Port=6
  Phase3_out0 : Outport  Port=7
  Phase3_out1 : Outport  Port=8
  Phase4_out0 : Outport  Port=9
  Phase4_out1 : Outport  Port=10
  Phase5_out0 : Outport  Port=11
  Phase5_out1 : Outport  Port=12
  Phase6_out0 : Outport  Port=13
  Phase6_out1 : Outport  Port=14
  Phase7_out0 : Outport  Port=15
  Phase7_out1 : Outport  Port=16
  wires:
  filter62/1 -> filter63/3
  filter1/1 -> filter2/3
  filter41/1 -> filter49/3
  filter6/1 -> filter7/3
  filter44/1 -> filter55/3
  filter17/1 -> filter24/3
  filter33/1 -> filter44/3
  filter50/1 -> filter51/3
  filter37/1 -> filter36/3
  filter36/1 -> filter35/3
  filter63/1 -> filter37/3
  filter10/1 -> filter9/3
  filter47/1 -> filter48/3
  filter52/1 -> filter53/3
  filter49/1 -> filter50/3
  filter12/1 -> filter11/3
  filter26/1 -> filter27/3
  filter25/1 -> filter26/3
  filter38/1 -> filter39/3
  filter59/1 -> filter60/3
  filter24/1 -> filter25/3
  filter32/1 -> filter33/3
  filter27/1 -> filter28/3
  filter13/1 -> filter12/3
  filter34/1 -> filter38/3
  filter19/1 -> filter18/3
  filter11/1 -> filter10/3
  filter2/1 -> filter3/3
  filter51/1 -> filter52/3
  filter40/1 -> filter41/3
  filter60/1 -> filter61/3
  filter5/1 -> filter6/3
  filter35/1 -> filter34/3
  filter45/1 -> filter43/3
  filter43/1 -> filter42/3
  filter58/1 -> filter59/3
  filter28/1 -> filter29/3
  filter18/1 -> filter22/3
  filter57/1 -> filter45/3
  filter30/1 -> filter31/3
  filter55/1 -> filter58/3
  filter53/1 -> filter54/3
  filter46/1 -> filter47/3
  filter3/1 -> filter4/3
  filter9/1 -> filter14/3
  filter14/1 -> filter15/3
  filter8/1 -> filter13/3
  filter21/1 -> filter20/3
  filter42/1 -> filter46/3
  filter16/1 -> filter17/3
  filter20/1 -> filter19/3
  filter31/1 -> filter21/3
  filter4/1 -> filter5/3
  filter56/1 -> filter57/3
  filter22/1 -> filter23/3
  filter/1 -> filter1/3
  filter48/1 -> PLIO/1
  PLIO/1 -> Phase7_out0/1
  filter48/2 -> PLIO1/1
  PLIO1/1 -> Phase7_out1/1
  filter39/1 -> PLIO2/1
  PLIO2/1 -> Phase5_out0/1
  filter39/2 -> PLIO3/1
  PLIO3/1 -> Phase5_out1/1
  filter23/1 -> PLIO4/1
  PLIO4/1 -> Phase3_out0/1
  filter23/2 -> PLIO5/1
  PLIO5/1 -> Phase3_out1/1
  filter15/1 -> PLIO6/1
  PLIO6/1 -> Phase1_out0/1
  filter15/2 -> PLIO7/1
  PLIO7/1 -> Phase1_out1/1
  P0_S0/1 -> PLIO8/1
  P0_S1/1 -> PLIO9/1
  PLIO8/1 -> FIFO15_1/1, FIFO23_1/1, FIFO39_1/1, FIFO48_1/1, FIFO0_1/1, FIFO16_1/1, FIFO32_1/1, FIFO40_1/1
  PLIO9/1 -> FIFO15_2/1, FIFO23_2/1, FIFO39_2/1, FIFO48_2/1, FIFO0_2/1, FIFO16_2/1, FIFO32_2/1, FIFO40_2/1
  P1_S0/1 -> PLIO12/1
  P1_S1/1 -> PLIO13/1
  PLIO12/1 -> FIFO38_1/1, FIFO47_1/1, FIFO14_1/1, FIFO22_1/1, FIFO1_1/1, FIFO17_1/1, FIFO33_1/1, FIFO41_1/1
  PLIO13/1 -> FIFO38_2/1, FIFO47_2/1, FIFO14_2/1, FIFO22_2/1, FIFO1_2/1, FIFO17_2/1, FIFO33_2/1, FIFO41_2/1
  P2_S0/1 -> PLIO16/1
  P2_S1/1 -> PLIO17/1
  PLIO16/1 -> FIFO9_1/1, FIFO18_1/1, FIFO34_1/1, FIFO46_1/1, FIFO24_1/1, FIFO49_1/1, FIFO44_1/1, FIFO2_1/1
  PLIO17/1 -> FIFO9_2/1, FIFO18_2/1, FIFO34_2/1, FIFO46_2/1, FIFO2_2/1, FIFO24_2/1, FIFO49_2/1, FIFO44_2/1
  P3_S0/1 -> PLIO20/1
  P3_S1/1 -> PLIO21/1
  PLIO20/1 -> FIFO10_1/1, FIFO19_1/1, FIFO35_1/1, FIFO42_1/1, FIFO3_1/1, FIFO25_1/1, FIFO55_1/1, FIFO50_1/1
  PLIO21/1 -> FIFO10_2/1, FIFO19_2/1, FIFO35_2/1, FIFO42_2/1, FIFO25_2/1, FIFO55_2/1, FIFO50_2/1, FIFO3_2/1
  P4_S0/1 -> PLIO24/1
  P4_S1/1 -> PLIO25/1
  PLIO24/1 -> FIFO20_1/1, FIFO36_1/1, FIFO43_1/1, FIFO11_1/1, FIFO4_1/1, FIFO26_1/1, FIFO58_1/1, FIFO51_1/1
  PLIO25/1 -> FIFO11_2/1, FIFO20_2/1, FIFO36_2/1, FIFO43_2/1, FIFO4_2/1, FIFO26_2/1, FIFO58_2/1, FIFO51_2/1
  P5_S0/1 -> PLIO28/1
  P5_S1/1 -> PLIO29/1
  PLIO28/1 -> FIFO5_1/1, FIFO27_1/1, FIFO59_1/1, FIFO52_1/1, FIFO21_1/1, FIFO37_1/1, FIFO45_1/1, FIFO12_1/1
  PLIO29/1 -> FIFO45_2/1, FIFO12_2/1, FIFO21_2/1, FIFO37_2/1, FIFO27_2/1, FIFO59_2/1, FIFO52_2/1, FIFO5_2/1
  P6_S0/1 -> PLIO32/1
  P6_S1/1 -> PLIO33/1
  PLIO32/1 -> FIFO13_1/1, FIFO31_1/1, FIFO63_1/1, FIFO57_1/1, FIFO6_1/1, FIFO28_1/1, FIFO60_1/1, FIFO53_1/1
  PLIO33/1 -> FIFO63_2/1, FIFO57_2/1, FIFO31_2/1, FIFO13_2/1, FIFO6_2/1, FIFO28_2/1, FIFO60_2/1, FIFO53_2/1
  P7_S0/1 -> PLIO36/1
  P7_S1/1 -> PLIO37/1
  PLIO36/1 -> FIFO62_1/1, FIFO56_1/1, FIFO30_1/1, FIFO8_1/1, FIFO7_1/1, FIFO29_1/1, FIFO54_1/1, FIFO61_1/1
  PLIO37/1 -> FIFO56_2/1, FIFO62_2/1, FIFO30_2/1, FIFO8_2/1, FIFO7_2/1, FIFO54_2/1, FIFO61_2/1, FIFO29_2/1
  filter7/1 -> PLIO40/1
  PLIO40/1 -> Phase0_out0/1
  filter7/2 -> PLIO41/1
  PLIO41/1 -> Phase0_out1/1
  filter29/2 -> PLIO42/1
  PLIO42/1 -> Phase2_out1/1
  filter29/1 -> PLIO43/1
  PLIO43/1 -> Phase2_out0/1
  filter61/2 -> PLIO44/1
  PLIO44/1 -> Phase4_out1/1
  filter61/1 -> PLIO45/1
  PLIO45/1 -> Phase4_out0/1
  filter54/2 -> PLIO46/1
  PLIO46/1 -> Phase6_out1/1
  filter54/1 -> PLIO47/1
  PLIO47/1 -> Phase6_out0/1
  FIFO40_1/1 -> filter40/1
  FIFO40_2/1 -> filter40/2
  FIFO32_1/1 -> filter32/1
  FIFO32_2/1 -> filter32/2
  FIFO16_1/1 -> filter16/1
  FIFO16_2/1 -> filter16/2
  FIFO0_1/1 -> filter/1
  FIFO0_2/1 -> filter/2
  FIFO48_1/1 -> filter48/1
  FIFO48_2/1 -> filter48/2
  FIFO39_1/1 -> filter39/1
  FIFO39_2/1 -> filter39/2
  FIFO23_1/1 -> filter23/1
  FIFO23_2/1 -> filter23/2
  FIFO15_1/1 -> filter15/1
  FIFO15_2/1 -> filter15/2
  FIFO41_1/1 -> filter41/1
  FIFO41_2/1 -> filter41/2
  FIFO33_1/1 -> filter33/1
  FIFO33_2/1 -> filter33/2
  FIFO17_1/1 -> filter17/1
  FIFO17_2/1 -> filter17/2
  FIFO1_1/1 -> filter1/1
  FIFO1_2/1 -> filter1/2
  FIFO47_1/1 -> filter47/1
  FIFO47_2/1 -> filter47/2
  FIFO38_1/1 -> filter38/1
  FIFO38_2/1 -> filter38/2
  FIFO22_1/1 -> filter22/1
  FIFO22_2/1 -> filter22/2
  FIFO14_1/1 -> filter14/1
  FIFO14_2/1 -> filter14/2
  FIFO49_1/1 -> filter49/1
  FIFO49_2/1 -> filter49/2
  FIFO44_1/1 -> filter44/1
  FIFO44_2/1 -> filter44/2
  FIFO24_1/1 -> filter24/1
  FIFO24_2/1 -> filter24/2
  FIFO2_1/1 -> filter2/1
  FIFO2_2/1 -> filter2/2
  FIFO46_1/1 -> filter46/1
  FIFO46_2/1 -> filter46/2
  FIFO34_1/1 -> filter34/1
  FIFO34_2/1 -> filter34/2
  FIFO18_1/1 -> filter18/1
  FIFO18_2/1 -> filter18/2
  FIFO9_1/1 -> filter9/1
  FIFO9_2/1 -> filter9/2
  FIFO50_1/1 -> filter50/1
  FIFO50_2/1 -> filter50/2
  FIFO55_1/1 -> filter55/1
  FIFO55_2/1 -> filter55/2
  FIFO25_1/1 -> filter25/1
  FIFO25_2/1 -> filter25/2
  FIFO3_1/1 -> filter3/1
  FIFO3_2/1 -> filter3/2
  FIFO42_1/1 -> filter42/1
  FIFO42_2/1 -> filter42/2
  FIFO35_1/1 -> filter35/1
  FIFO35_2/1 -> filter35/2
  FIFO19_1/1 -> filter19/1
  FIFO19_2/1 -> filter19/2
  FIFO10_1/1 -> filter10/1
  FIFO10_2/1 -> filter10/2
  FIFO51_1/1 -> filter51/1
  FIFO51_2/1 -> filter51/2
  FIFO58_1/1 -> filter58/1
  FIFO58_2/1 -> filter58/2
  FIFO26_1/1 -> filter26/1
  FIFO26_2/1 -> filter26/2
  FIFO4_1/1 -> filter4/1
  FIFO4_2/1 -> filter4/2
  FIFO43_1/1 -> filter43/1
  FIFO43_2/1 -> filter43/2
  FIFO36_1/1 -> filter36/1
  FIFO36_2/1 -> filter36/2
  FIFO20_1/1 -> filter20/1
  FIFO20_2/1 -> filter20/2
  FIFO11_1/1 -> filter11/1
  FIFO11_2/1 -> filter11/2
  FIFO52_1/1 -> filter52/1
  FIFO52_2/1 -> filter52/2
  FIFO59_1/1 -> filter59/1
  FIFO59_2/1 -> filter59/2
  FIFO27_1/1 -> filter27/1
  FIFO27_2/1 -> filter27/2
  FIFO5_1/1 -> filter5/1
  FIFO5_2/1 -> filter5/2
  FIFO45_1/1 -> filter45/1
  FIFO45_2/1 -> filter45/2
  FIFO37_1/1 -> filter37/1
  FIFO37_2/1 -> filter37/2
  FIFO21_1/1 -> filter21/1
  FIFO21_2/1 -> filter21/2
  FIFO12_1/1 -> filter12/1
  FIFO12_2/1 -> filter12/2
  FIFO53_1/1 -> filter53/1
  FIFO53_2/1 -> filter53/2
  FIFO60_1/1 -> filter60/1
  FIFO60_2/1 -> filter60/2
  FIFO28_1/1 -> filter28/1
  FIFO28_2/1 -> filter28/2
  FIFO6_1/1 -> filter6/1
  FIFO6_2/1 -> filter6/2
  FIFO57_1/1 -> filter57/1
  FIFO57_2/1 -> filter57/2
  FIFO63_1/1 -> filter63/1
  FIFO63_2/1 -> filter63/2
  FIFO31_1/1 -> filter31/1
  FIFO31_2/1 -> filter31/2
  FIFO13_1/1 -> filter13/1
  FIFO13_2/1 -> filter13/2
  FIFO54_1/1 -> filter54/1
  FIFO54_2/1 -> filter54/2
  FIFO61_1/1 -> filter61/1
  FIFO61_2/1 -> filter61/2
  FIFO29_1/1 -> filter29/1
  FIFO29_2/1 -> filter29/2
  FIFO7_1/1 -> filter7/1
  FIFO7_2/1 -> filter7/2
  FIFO56_1/1 -> filter56/1
  FIFO56_2/1 -> filter56/2
  FIFO62_1/1 -> filter62/1
  FIFO62_2/1 -> filter62/2
  FIFO30_1/1 -> filter30/1
  FIFO30_2/1 -> filter30/2
  FIFO8_1/1 -> filter8/1
  FIFO8_2/1 -> filter8/2
